simulink model "Maq_Sincronica"  (R2020a)
settings: Solver=VariableStepAuto  StartTime=0.0  StopTime=5  MaxStep=10e-4  RelTol=1e-3
values from neighbouring files (symbols this model uses):
  delto = delt    [ParamV2.m]    (also in Parametros.m)
  Domega = 0    [ParamV2.m]    (also in Parametros.m)
  H = 3.77    [ParamV2.m]    (also in Parametros.m)
  Psido = 1    [ParamV2.m]    (also in Parametros.m = xls*(-Ido) + Psiado)
  Psifo = 1    [ParamV2.m]    (also in Parametros.m = xplf*Ifo + Psiado)
  Psikdo = Psiado    (= 1)    [ParamV2.m]    (also in Parametros.m = Psiado)
  Psikqo = Psiaqo    (= 0)    [ParamV2.m]    (also in Parametros.m = Psiaqo)
  Psiqo = 0    [ParamV2.m]    (also in Parametros.m = xls*(-Iqo) + Psiaqo)
  rpf = rpf/Zbase    [ParamV2.m]    (also in Parametros.m = 0.000580431542227)
  rpkd = rpkd/Zbase    [ParamV2.m]    (also in Parametros.m = 0.0203088338841)
  rpkq = rpkq/Zbase    [ParamV2.m]    (also in Parametros.m = 0.0727096597855)
  rs = rs/Zbase    [ParamV2.m]    (also in Parametros.m = 0.0048)
  tef_time = [0 tstop]    [ParamV2.m]    (also in Parametros.m = [0 0.5 3 tstop])
  tef_value = [1 1]*Efo    [ParamV2.m]    (also in Parametros.m = [1  1  1 1]*ef)
  thetaro = delto+thetaeo    [ParamV2.m]    (also in Parametros.m)
  tmech_time = [4 5.5 5.5 7.5 7.5 tstop]    [ParamV2.m]    (also in Parametros.m = [0  0.5  0.5  3  3  tstop])
  tmech_value = [1 1 0 0 -1 -1]*Tmech    [ParamV2.m]    (also in Parametros.m = [1  1  0  0  -1  -1]*Tmech)
  Vm = 120*sqrt(2)    [ParamV2.m]    (also in Parametros.m = abs(Vt))
  wb = wbase    (= 376.991118431)    [ParamV2.m]    (also in Parametros.m)
  xls = xls/Zbase    [ParamV2.m]    (also in Parametros.m = 0.215)
  xmd = xmd/Zbase    [ParamV2.m]    (also in Parametros.m = 1.575)
  xMD = (1/xls + 1/xmd + 1/xplf + 1/xplkd)^(-1)    (= 0.0469090909091)    [ParamV2.m]    (also in Parametros.m)
  xMQ = (1/xls + 1/xmq + 1/xplkq)^(-1)    (= 0.0469090909091)    [ParamV2.m]    (also in Parametros.m)
  xplf = xplf/Zbase    [ParamV2.m]    (also in Parametros.m = 0.153658536585)
  xplkd = xplkd/Zbase    [ParamV2.m]    (also in Parametros.m = 0.105)
  xplkq = xplkq/Zbase    [ParamV2.m]    (also in Parametros.m = 0.0625992779783)
settings Model: Creator=jschi  LastModifiedBy=pc

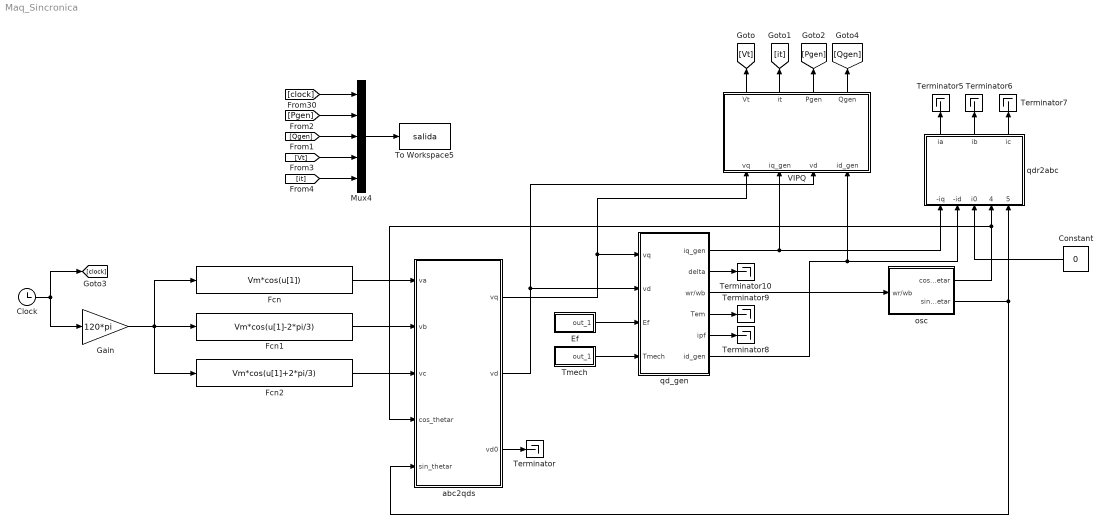
== system Maq_Sincronica ==
  Clock : Clock
  Constant : Constant  Value=0
  Ef : Subsystem  mask(Repeating table){rep_seq_t=tef_time, rep_seq_y=tef_value}
      mask prompts: rep_seq_t "Time values:"; rep_seq_y "Output values:"
      mask help: Repeating table.
      mask init:
      | period = max(rep_seq_t);
      mask Help: Repeats cycle given in table. Time values should be monotonically increasing.
      mask Display: plot([rep_seq_t,rep_seq_t+period,rep_seq_t+2*period,rep_seq_t(1)+3*period],[rep_seq_y,rep_seq_y,rep_seq_y,rep_seq_y(1)])
  Fcn : Fcn  Expr=Vm*cos(u[1])
  Fcn1 : Fcn  Expr=Vm*cos(u[1]-2*pi/3)
  Fcn2 : Fcn  Expr=Vm*cos(u[1]+2*pi/3)
  Gain : Gain  Gain=120*pi
  Mux4 : Mux  Inputs=5
  Terminator{,5..10} (7 alike) : Terminator
  Tmech : Subsystem  mask(Repeating table){rep_seq_t=tmech_time, rep_seq_y=tmech_value}
      mask prompts: rep_seq_t "Time values:"; rep_seq_y "Output values:"
      mask help: Repeating table.
      mask init:
      | period = max(rep_seq_t);
      mask Help: Repeats cycle given in table. Time values should be monotonically increasing.
      mask Display: plot([rep_seq_t,rep_seq_t+period,rep_seq_t+2*period,rep_seq_t(1)+3*period],[rep_seq_y,rep_seq_y,rep_seq_y,rep_seq_y(1)])
  To Workspace5 : ToWorkspace  VariableName=salida  SampleTime=-1
  VIPQ : Subsystem
  abc2qds : Subsystem
  osc : Subsystem
  qd_gen : Subsystem
  qdr2abc : Subsystem
  wires:
  Fcn/1 -> abc2qds/1(va)
  Gain/1 -> Fcn2/1, Fcn1/1, Fcn/1
  Fcn1/1 -> abc2qds/2(vb)
  Fcn2/1 -> abc2qds/3(vc)
  Clock/1 -> [clock], Gain/1
  Tmech/1(out_1) -> qd_gen/4(Tmech)
  qd_gen/3(wr/wb) -> osc/1(wr/wb)
  osc/1(cos_thetar) -> qdr2abc/4(cos_thetar), abc2qds/4(cos_thetar)
  osc/2(sin_thetar) -> abc2qds/5(sin_thetar), qdr2abc/5(sin_thetar)
  qd_gen/6(id_gen) -> qdr2abc/2(-id), VIPQ/4(id_gen)
  qd_gen/1(iq_gen) -> qdr2abc/1(-iq), VIPQ/2(iq_gen)
  abc2qds/1(vq) -> qd_gen/1(vq), VIPQ/1(vq)
  abc2qds/2(vd) -> qd_gen/2(vd), VIPQ/3(vd)
  abc2qds/3(vd0) -> Terminator/1
  Ef/1(out_1) -> qd_gen/3(Ef)
  [Pgen] -> Mux4/2
  [it] -> Mux4/5
  Mux4/1 -> To Workspace5/1
  [Vt] -> Mux4/4
  [clock] -> Mux4/1
  [Qgen] -> Mux4/3
  VIPQ/1(Vt) -> [Vt]
  qdr2abc/1(ia) -> Terminator5/1
  qdr2abc/2(ib) -> Terminator6/1
  qdr2abc/3(ic) -> Terminator7/1
  Constant/1 -> qdr2abc/3(i0)
  qd_gen/5(ipf) -> Terminator8/1
  qd_gen/4(Tem) -> Terminator9/1
  qd_gen/2(delta) -> Terminator10/1
  VIPQ/2(it) -> [it]
  VIPQ/3(Pgen) -> [Pgen]
  VIPQ/4(Qgen) -> [Qgen]

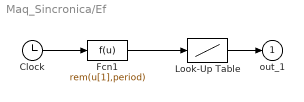
== system Maq_Sincronica/Ef ==
  Clock : Clock
  Fcn1 : Fcn  Expr=rem(u[1],period)
  Look-Up Table : Lookup  InputValues=rep_seq_t  Table=rep_seq_y  SaturateOnIntegerOverflow=on
  out_1 : Outport  InitialOutput=0
  wires:
  Look-Up Table/1 -> out_1/1
  Clock/1 -> Fcn1/1
  Fcn1/1 -> Look-Up Table/1

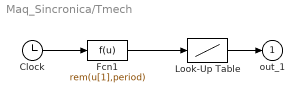
== system Maq_Sincronica/Tmech ==
  Clock : Clock
  Fcn1 : Fcn  Expr=rem(u[1],period)
  Look-Up Table : Lookup  InputValues=rep_seq_t  Table=rep_seq_y  SaturateOnIntegerOverflow=on
  out_1 : Outport  InitialOutput=0
  wires:
  Look-Up Table/1 -> out_1/1
  Clock/1 -> Fcn1/1
  Fcn1/1 -> Look-Up Table/1

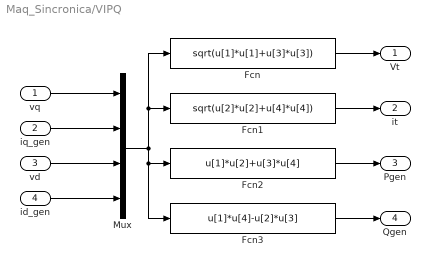
== system Maq_Sincronica/VIPQ ==
  vq : Inport
  iq_gen : Inport  Port=2
  vd : Inport  Port=3
  id_gen : Inport  Port=4
  Fcn : Fcn  Expr=sqrt(u[1]*u[1]+u[3]*u[3])
  Fcn1 : Fcn  Expr=sqrt(u[2]*u[2]+u[4]*u[4])
  Fcn2 : Fcn  Expr=u[1]*u[2]+u[3]*u[4]
  Fcn3 : Fcn  Expr=u[1]*u[4]-u[2]*u[3]
  Mux : Mux
  Vt : Outport
  it : Outport  Port=2
  Pgen : Outport  Port=3
  Qgen : Outport  Port=4
  wires:
  vd/1 -> Mux/3
  iq_gen/1 -> Mux/2
  vq/1 -> Mux/1
  Mux/1 -> Fcn1/1, Fcn/1, Fcn3/1, Fcn2/1
  Fcn3/1 -> Qgen/1
  Fcn2/1 -> Pgen/1
  Fcn1/1 -> it/1
  Fcn/1 -> Vt/1
  id_gen/1 -> Mux/4

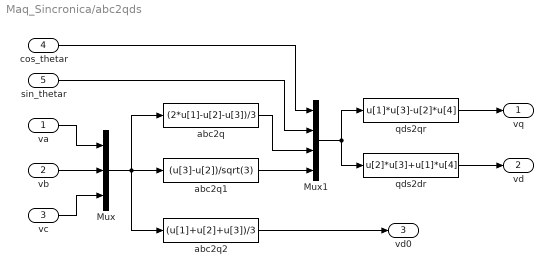
== system Maq_Sincronica/abc2qds ==
  va : Inport
  vb : Inport  Port=2
  vc : Inport  Port=3
  cos_thetar : Inport  Port=4
  sin_thetar : Inport  Port=5
  Mux : Mux  Inputs=3
  Mux1 : Mux
  abc2q : Fcn  Expr=(2*u[1]-u[2]-u[3])/3
  abc2q1 : Fcn  Expr=(u[3]-u[2])/sqrt(3)
  abc2q2 : Fcn  Expr=(u[1]+u[2]+u[3])/3
  qds2dr : Fcn  Expr=u[2]*u[3]+u[1]*u[4]
  qds2qr : Fcn  Expr=u[1]*u[3]-u[2]*u[4]
  vq : Outport
  vd : Outport  Port=2
  vd0 : Outport  Port=3
  wires:
  va/1 -> Mux/1
  vb/1 -> Mux/2
  vc/1 -> Mux/3
  Mux/1 -> abc2q2/1, abc2q1/1, abc2q/1
  abc2q1/1 -> Mux1/4
  abc2q/1 -> Mux1/3
  sin_thetar/1 -> Mux1/2
  cos_thetar/1 -> Mux1/1
  abc2q2/1 -> vd0/1
  Mux1/1 -> qds2dr/1, qds2qr/1
  qds2qr/1 -> vq/1
  qds2dr/1 -> vd/1

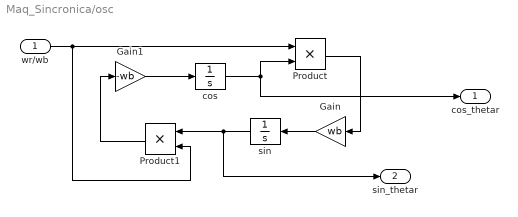
== system Maq_Sincronica/osc ==
  wr/wb : Inport
  Gain : Gain  Gain=wb
  Gain1 : Gain  Gain=-wb
  Product : Product
  Product1 : Product
  cos : Integrator  InitialCondition=cos(thetaro)
  sin : Integrator  InitialCondition=sin(thetaro)
  cos_thetar : Outport
  sin_thetar : Outport  Port=2
  wires:
  sin/1 -> sin_thetar/1, Product1/1
  cos/1 -> cos_thetar/1, Product/2
  wr/wb/1 -> Product/1, Product1/2
  Product/1 -> Gain/1
  Gain/1 -> sin/1
  Gain1/1 -> cos/1
  Product1/1 -> Gain1/1

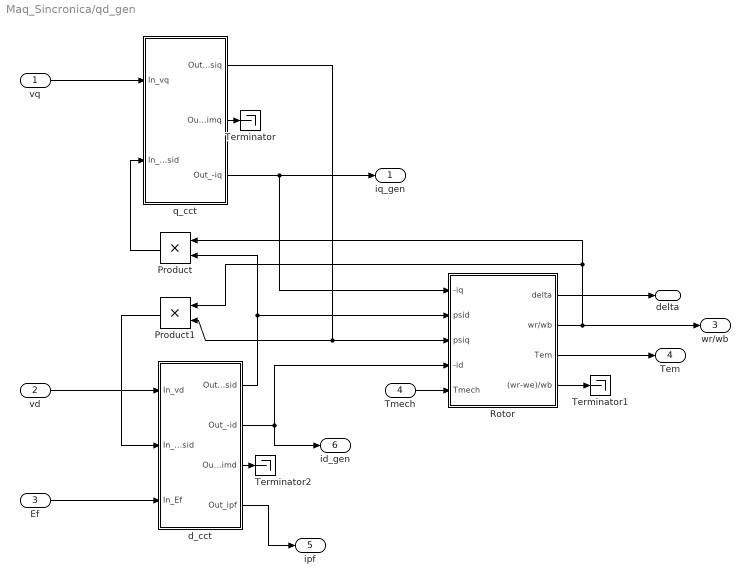
== system Maq_Sincronica/qd_gen ==
  vq : Inport
  vd : Inport  Port=2
  Ef : Inport  Port=3
  Tmech : Inport  Port=4
  Product : Product
  Product1 : Product
  Rotor : Subsystem
  Terminator : Terminator
  Terminator1 : Terminator
  Terminator2 : Terminator
  d_cct : Subsystem
  q_cct : Subsystem
  iq_gen : Outport
  delta : Outport  Port=2
  wr/wb : Outport  Port=3
  Tem : Outport  Port=4
  ipf : Outport  Port=5
  id_gen : Outport  Port=6
  wires:
  Tmech/1 -> Rotor/5(Tmech)
  vq/1 -> q_cct/1(In_vq)
  Product/1 -> q_cct/2(In_wrpsid)
  q_cct/1(Out_psiq) -> Rotor/3(psiq), Product1/2
  q_cct/3(Out_-iq) -> iq_gen/1, Rotor/1(-iq)
  q_cct/2(Out_psimq) -> Terminator/1
  Product1/1 -> d_cct/2(In_wrpsid)
  vd/1 -> d_cct/1(In_vd)
  Ef/1 -> d_cct/3(In_Ef)
  d_cct/4(Out_ipf) -> ipf/1
  d_cct/2(Out_-id) -> Rotor/4(-id), id_gen/1
  d_cct/1(Out_psid) -> Product/2, Rotor/2(psid)
  Rotor/3(Tem) -> Tem/1
  Rotor/1(delta) -> delta/1
  Rotor/2(wr/wb) -> Product/1, Product1/1, wr/wb/1
  Rotor/4((wr-we)/wb) -> Terminator1/1
  d_cct/3(Out_psimd) -> Terminator2/1

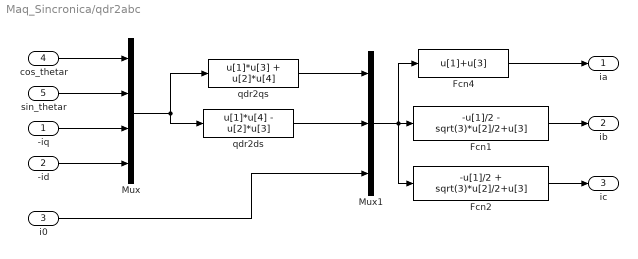
== system Maq_Sincronica/qdr2abc ==
  -iq : Inport
  -id : Inport  Port=2
  i0 : Inport  Port=3
  cos_thetar : Inport  Port=4
  sin_thetar : Inport  Port=5
  Fcn1 : Fcn  Expr=-u[1]/2 - sqrt(3)*u[2]/2+u[3]
  Fcn2 : Fcn  Expr=-u[1]/2 + sqrt(3)*u[2]/2+u[3]
  Fcn4 : Fcn  Expr=u[1]+u[3]
  Mux : Mux
  Mux1 : Mux  Inputs=3
  qdr2ds : Fcn  Expr=u[1]*u[4] - u[2]*u[3]
  qdr2qs : Fcn  Expr=u[1]*u[3] + u[2]*u[4]
  ia : Outport
  ib : Outport  Port=2
  ic : Outport  Port=3
  wires:
  sin_thetar/1 -> Mux/2
  cos_thetar/1 -> Mux/1
  Fcn1/1 -> ib/1
  Fcn2/1 -> ic/1
  Fcn4/1 -> ia/1
  Mux1/1 -> Fcn2/1, Fcn4/1, Fcn1/1
  Mux/1 -> qdr2qs/1, qdr2ds/1
  qdr2ds/1 -> Mux1/2
  qdr2qs/1 -> Mux1/1
  i0/1 -> Mux1/3
  -id/1 -> Mux/4
  -iq/1 -> Mux/3

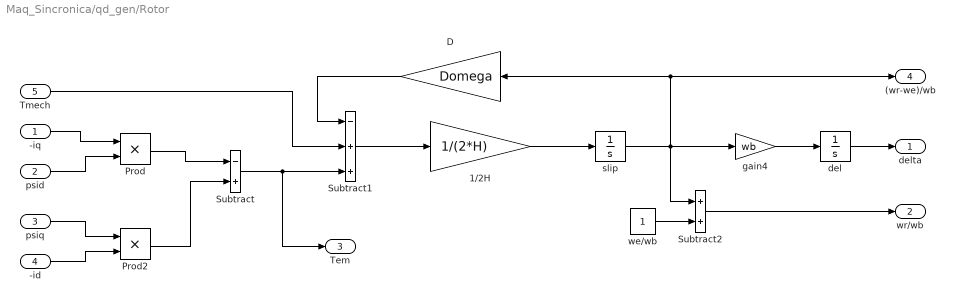
== system Maq_Sincronica/qd_gen/Rotor ==
  -iq : Inport
  psid : Inport  Port=2
  psiq : Inport  Port=3
  -id : Inport  Port=4
  Tmech : Inport  Port=5
  1/2H : Gain  Gain=1/(2*H)
  D : Gain  Gain=Domega
  Prod : Product
  Prod2 : Product
  Subtract : Sum  Inputs=-+
  Subtract1 : Sum  Inputs=-++
  Subtract2 : Sum
  del : Integrator  InitialCondition=delto
  gain4 : Gain  Gain=wb
  slip : Integrator
  we/wb : Constant
  delta : Outport
  wr/wb : Outport  Port=2
  Tem : Outport  Port=3
  (wr-we)/wb : Outport  Port=4
  wires:
  psid/1 -> Prod/2
  -iq/1 -> Prod/1
  Prod/1 -> Subtract/1
  psiq/1 -> Prod2/1
  -id/1 -> Prod2/2
  Prod2/1 -> Subtract/2
  Subtract1/1 -> 1/2H/1
  1/2H/1 -> slip/1
  slip/1 -> gain4/1, (wr-we)/wb/1, D/1, Subtract2/1
  Subtract/1 -> Tem/1, Subtract1/3
  Tmech/1 -> Subtract1/2
  D/1 -> Subtract1/1
  we/wb/1 -> Subtract2/2
  Subtract2/1 -> wr/wb/1
  gain4/1 -> del/1
  del/1 -> delta/1

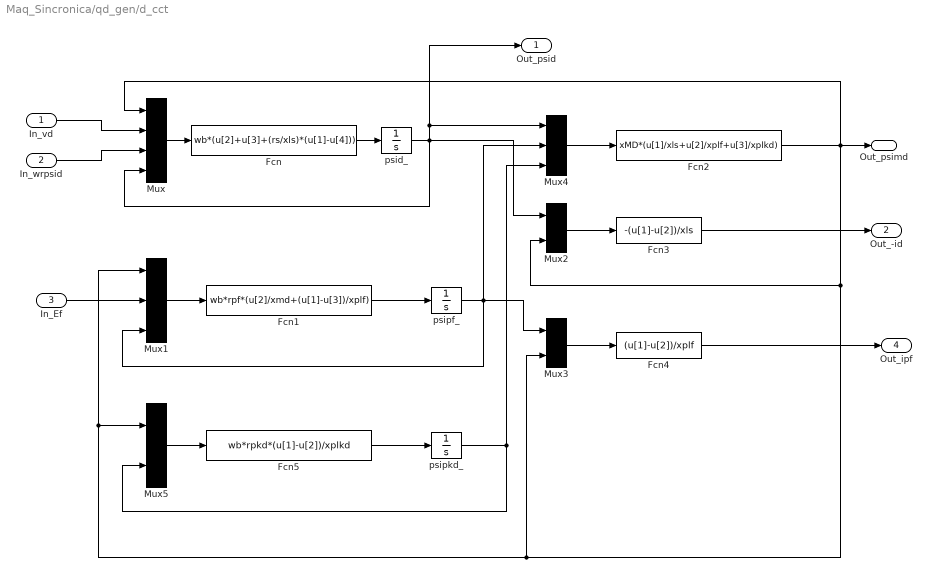
== system Maq_Sincronica/qd_gen/d_cct ==
  In_vd : Inport
  In_wrpsid : Inport  Port=2
  In_Ef : Inport  Port=3
  Fcn : Fcn  Expr=wb*(u[2]+u[3]+(rs/xls)*(u[1]-u[4]))
  Fcn1 : Fcn  Expr=wb*rpf*(u[2]/xmd+(u[1]-u[3])/xplf)
  Fcn2 : Fcn  Expr=xMD*(u[1]/xls+u[2]/xplf+u[3]/xplkd)
  Fcn3 : Fcn  Expr=-(u[1]-u[2])/xls
  Fcn4 : Fcn  Expr=(u[1]-u[2])/xplf
  Fcn5 : Fcn  Expr=wb*rpkd*(u[1]-u[2])/xplkd
  Mux : Mux
  Mux1 : Mux  Inputs=3
  Mux2 : Mux  Inputs=2
  Mux3 : Mux  Inputs=2
  Mux4 : Mux  Inputs=3
  Mux5 : Mux  Inputs=2
  psid_ : Integrator  InitialCondition=Psido
  psipf_ : Integrator  InitialCondition=Psifo
  psipkd_ : Integrator  InitialCondition=Psikdo
  Out_psid : Outport
  Out_-id : Outport  Port=2
  Out_psimd : Outport  Port=3
  Out_ipf : Outport  Port=4
  wires:
  Mux/1 -> Fcn/1
  In_vd/1 -> Mux/2
  Mux1/1 -> Fcn1/1
  Fcn1/1 -> psipf_/1
  Fcn/1 -> psid_/1
  psid_/1 -> Mux/4, Mux2/1, Mux4/1, Out_psid/1
  In_wrpsid/1 -> Mux/3
  Mux4/1 -> Fcn2/1
  Mux2/1 -> Fcn3/1
  Mux3/1 -> Fcn4/1
  Mux5/1 -> Fcn5/1
  Fcn5/1 -> psipkd_/1
  In_Ef/1 -> Mux1/2
  psipkd_/1 -> Mux5/2, Mux4/3
  psipf_/1 -> Mux4/2, Mux1/3, Mux3/1
  Fcn4/1 -> Out_ipf/1
  Fcn3/1 -> Out_-id/1
  Fcn2/1 -> Mux5/1, Mux1/1, Mux3/2, Mux2/2, Out_psimd/1, Mux/1

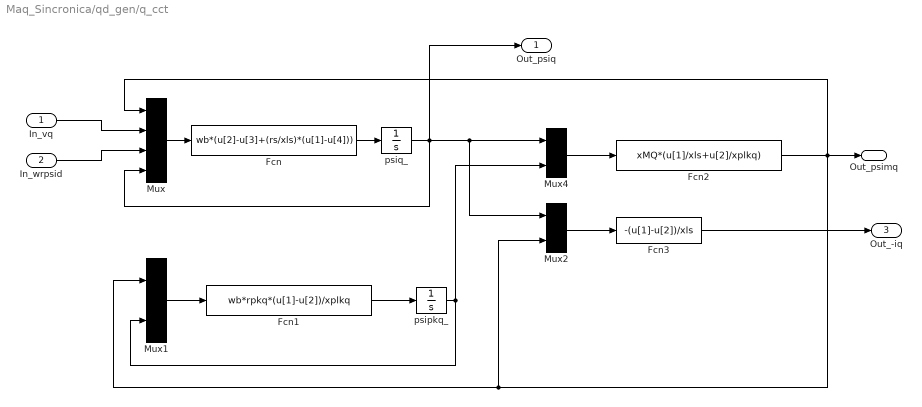
== system Maq_Sincronica/qd_gen/q_cct ==
  In_vq : Inport
  In_wrpsid : Inport  Port=2
  Fcn : Fcn  Expr=wb*(u[2]-u[3]+(rs/xls)*(u[1]-u[4]))
  Fcn1 : Fcn  Expr=wb*rpkq*(u[1]-u[2])/xplkq
  Fcn2 : Fcn  Expr=xMQ*(u[1]/xls+u[2]/xplkq)
  Fcn3 : Fcn  Expr=-(u[1]-u[2])/xls
  Mux : Mux
  Mux1 : Mux  Inputs=2
  Mux2 : Mux  Inputs=2
  Mux4 : Mux  Inputs=2
  psipkq_ : Integrator  InitialCondition=Psikqo
  psiq_ : Integrator  InitialCondition=Psiqo
  Out_psiq : Outport
  Out_psimq : Outport  Port=2
  Out_-iq : Outport  Port=3
  wires:
  Mux/1 -> Fcn/1
  In_vq/1 -> Mux/2
  Mux1/1 -> Fcn1/1
  Fcn1/1 -> psipkq_/1
  Fcn/1 -> psiq_/1
  psiq_/1 -> Mux/4, Out_psiq/1, Mux2/1, Mux4/1
  psipkq_/1 -> Mux1/2, Mux4/2
  In_wrpsid/1 -> Mux/3
  Mux4/1 -> Fcn2/1
  Mux2/1 -> Fcn3/1
  Fcn2/1 -> Mux2/2, Mux1/1, Mux/1, Out_psimq/1
  Fcn3/1 -> Out_-iq/1
